simulink model "propagationSimulator"  (R2020a)
settings: Solver=VariableStepAuto  StartTime=0.0  StopTime=inf  RelTol=1e-3
InitFcn:
  | initData
values from neighbouring files (symbols this model uses):
  L = 2    [initData.m]
  N = N1*N2    (= 50)    [initData.m]    (also in populationAnimator.m = size(obj.Data.Status, 2); propagationAnimator.m = size(obj.Data.Status, 2))
  R = 0.02    [initData.m]    (also in populationAnimator.m = obj.Radius; propagationAnimator.m = obj.Radius)
  state0 = zeros(N,1)    [initData.m]
  W = 1    [initData.m]
undefined symbols (not defined in the file or in its folder): DiscIntNeverNeededParam, healTime, immobilized, pos0, v0
libraries: simulink x3
settings Model: SimulationMode=accelerator  PauseTimes=8.4  PacingRate=2  OrderedModelArguments=off  Creator=guy  LastModifiedBy=Pavel Roslovets
settings SolverCC: ZeroCrossAlgorithm=Adaptive
settings DataIOCC: MaxDataPoints=1
settings DebuggingCC: ReadBeforeWriteMsg=DisableAll  WriteAfterWriteMsg=DisableAll  WriteAfterReadMsg=DisableAll  ArithmeticOperatorsInVariantConditions=warning
settings SFSimCC: SimUseLocalCustomCode=off  CustomCodeUndefinedFunction=UseInterfaceOnly
settings RTWCC: RTWUseLocalCustomCode=off

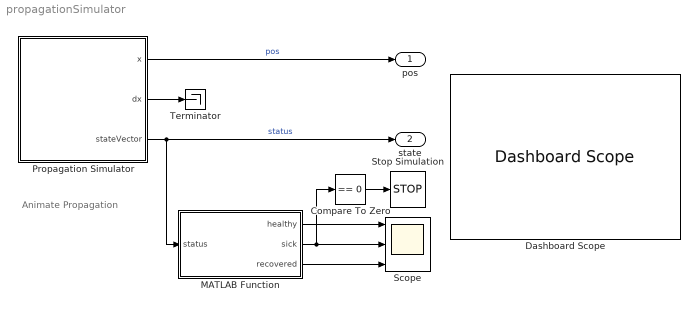
== system propagationSimulator ==
  note: Animate Propagation
  Compare To Zero : simulink/Logic and Bit Operations/Compare To Zero  relop===  OutDataTypeStr=boolean
  Dashboard Scope : DashboardScope  Ymin=0  Ymax=100
  MATLAB Function : MATLAB Function  TreatAsAtomicUnit=on
  Propagation Simulator : Stateflow chart  TreatAsAtomicUnit=on
  Scope : Scope  NumInputPorts=3
  Stop Simulation : Stop
  Terminator : Terminator
  pos : Outport  VectorParamsAs1DForOutWhenUnconnected=off
  state : Outport  Port=2  VectorParamsAs1DForOutWhenUnconnected=off
  wires:
  Propagation Simulator/1(x) -> pos/1  "pos"
  Propagation Simulator/2(dx) -> Terminator/1
  Compare To Zero/1 -> Stop Simulation/1
  MATLAB Function/1(healthy) -> Scope/1
  MATLAB Function/2(sick) -> Scope/2, Compare To Zero/1
  MATLAB Function/3(recovered) -> Scope/3
  Propagation Simulator/3(stateVector) -> state/1, MATLAB Function/1(status)  "status"

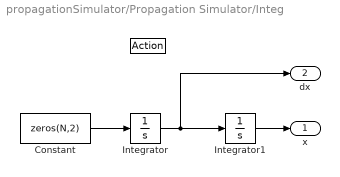
== system propagationSimulator/Propagation Simulator/Integ ==
  " " : ActionPort
      settings: CopyFcn=Stateflow.SLINSF.SimulinkMan.removeBlockPreDeleteFcn  PreDeleteFcn=Stateflow.SLINSF.SimulinkMan.unsafePredeleteFcn
  Constant : Constant  Value=zeros(N,2)
  Integrator : Integrator  ContinuousStateAttributes='dx0'
  Integrator1 : Integrator  ContinuousStateAttributes='x0'
  x : Outport  OutDataTypeStr=double  PortDimensions=[N 2]  VectorParamsAs1DForOutWhenUnconnected=off
  dx : Outport  Port=2  OutDataTypeStr=double  PortDimensions=[N 2]  VectorParamsAs1DForOutWhenUnconnected=off
  wires:
  Integrator1/1 -> x/1
  Constant/1 -> Integrator/1
  Integrator/1 -> dx/1, Integrator1/1

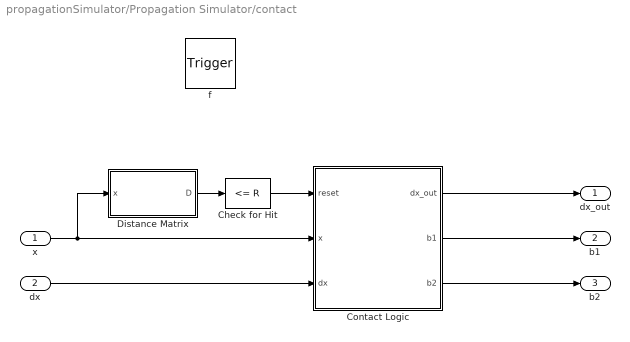
== system propagationSimulator/Propagation Simulator/contact ==
  x : Inport  OutDataTypeStr=double  PortDimensions=[N 2]
  dx : Inport  Port=2  OutDataTypeStr=double  PortDimensions=[N 2]
  f : TriggerPort  TriggerType=function-call  VariantControl=(inherit)
      settings: CopyFcn=Stateflow.SLINSF.SimulinkMan.removeBlockPreDeleteFcn  PreDeleteFcn=Stateflow.SLINSF.SimulinkMan.unsafePredeleteFcn
  Check for Hit : simulink/Logic and Bit Operations/Compare To Constant  relop=<=  const=R  OutDataTypeStr=boolean
  Contact Logic : Subsystem  TreatAsAtomicUnit=on
  Distance Matrix : Subsystem  TreatAsAtomicUnit=on
  dx_out : Outport  VectorParamsAs1DForOutWhenUnconnected=off
  b1 : Outport  Port=2
  b2 : Outport  Port=3
  wires:
  Check for Hit/1 -> Contact Logic/1(reset)
  x/1 -> Distance Matrix/1(x), Contact Logic/2(x)
  dx/1 -> Contact Logic/3(dx)
  Distance Matrix/1(D) -> Check for Hit/1
  Contact Logic/2(b1) -> b1/1
  Contact Logic/3(b2) -> b2/1
  Contact Logic/1(dx_out) -> dx_out/1

== system propagationSimulator/Propagation Simulator/heal ==
  stateIn : Inport  OutDataTypeStr=double  PortDimensions=N
  f : TriggerPort  TriggerType=function-call  VariantControl=(inherit)
      settings: CopyFcn=Stateflow.SLINSF.SimulinkMan.removeBlockPreDeleteFcn  PreDeleteFcn=Stateflow.SLINSF.SimulinkMan.unsafePredeleteFcn
  Compare To Constant2 : simulink/Logic and Bit Operations/Compare To Constant  relop=>=  const=healTime  OutDataTypeStr=boolean
  Discrete-Time Integrator : DiscreteIntegrator  SampleTime=-1  ICPrevOutput=DiscIntNeverNeededParam  ICPrevScaledInput=DiscIntNeverNeededParam
  MATLAB Function : MATLAB Function  TreatAsAtomicUnit=on
  stateVector : Outport
  wires:
  MATLAB Function/1(states) -> stateVector/1
  Discrete-Time Integrator/1 -> Compare To Constant2/1
  Compare To Constant2/1 -> MATLAB Function/2(immuned)
  stateIn/1 -> Discrete-Time Integrator/1, MATLAB Function/1("states ")

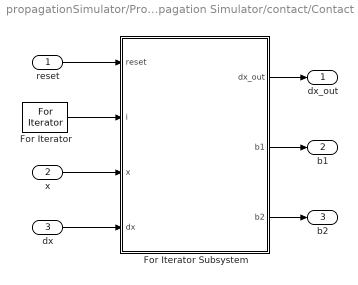
== system propagationSimulator/Propagation Simulator/contact/Contact Logic ==
  reset : Inport
  x : Inport  Port=2
  dx : Inport  Port=3
  For Iterator : ForIterator  ResetStates=reset  IterationLimit=N
  For Iterator Subsystem : Subsystem  TreatAsAtomicUnit=on
  dx_out : Outport  VectorParamsAs1DForOutWhenUnconnected=off
  b1 : Outport  Port=2
  b2 : Outport  Port=3
  wires:
  For Iterator Subsystem/1(dx_out) -> dx_out/1
  For Iterator/1 -> For Iterator Subsystem/2(i)
  reset/1 -> For Iterator Subsystem/1(reset)
  dx/1 -> For Iterator Subsystem/4(dx)
  x/1 -> For Iterator Subsystem/3(x)
  For Iterator Subsystem/2(b1) -> b1/1
  For Iterator Subsystem/3(b2) -> b2/1

== system propagationSimulator/Propagation Simulator/contact/Distance Matrix ==
  x : Inport
  For Iterator : ForIterator  ResetStates=reset  IterationLimit=N
  For Iterator Subsystem : Subsystem  TreatAsAtomicUnit=on
  D : Outport  VectorParamsAs1DForOutWhenUnconnected=off
  wires:
  For Iterator/1 -> For Iterator Subsystem/2(i)
  For Iterator Subsystem/1(Out1) -> D/1
  x/1 -> For Iterator Subsystem/1(x)

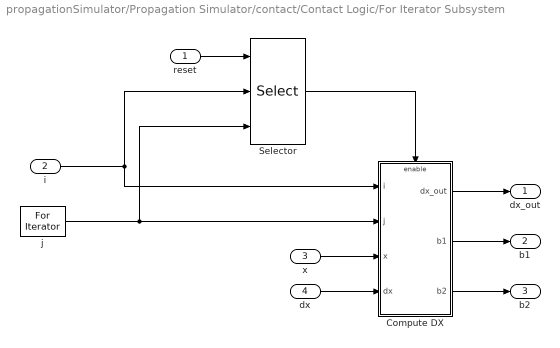
== system propagationSimulator/Propagation Simulator/contact/Contact Logic/For Iterator Subsystem ==
  reset : Inport
  i : Inport  Port=2
  x : Inport  Port=3
  dx : Inport  Port=4
  Compute DX : Subsystem
  Selector : Selector  NumberOfDimensions=2  InputPortWidth=3  IndexOptions=Index vector (port),Index vector (port)  Indices=[1 3],1  OutputSizes=1,1
  j : ForIterator  IterationLimit=N
  dx_out : Outport  VectorParamsAs1DForOutWhenUnconnected=off
  b1 : Outport  Port=2
  b2 : Outport  Port=3
  wires:
  reset/1 -> Selector/1
  j/1 -> Selector/3, Compute DX/2(j)
  i/1 -> Selector/2, Compute DX/1(i)
  Compute DX/1(dx_out) -> dx_out/1
  Selector/1 -> Compute DX/Enable
  dx/1 -> Compute DX/4(dx)
  x/1 -> Compute DX/3(x)
  Compute DX/2(b1) -> b1/1
  Compute DX/3(b2) -> b2/1

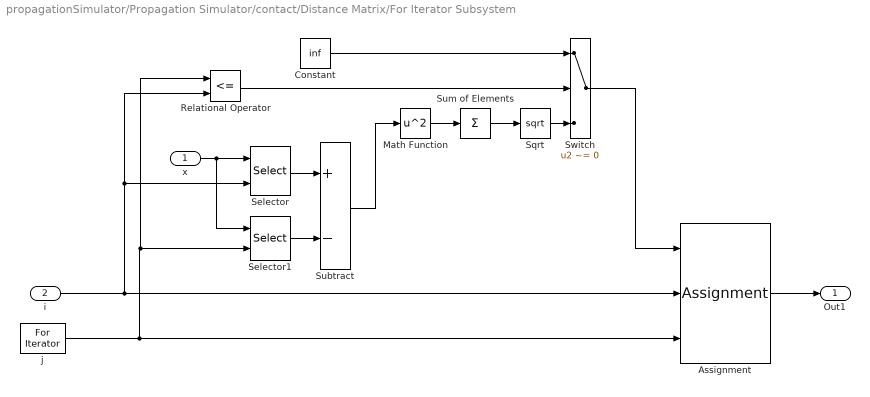
== system propagationSimulator/Propagation Simulator/contact/Distance Matrix/For Iterator Subsystem ==
  x : Inport
  i : Inport  Port=2
  Assignment : Assignment  NumberOfDimensions=2  OutputInitialize=Specify size for each dimension in table  IndexOptions=Index vector (port),Index vector (port)  Indices=1,1  OutputSizes=N,N
  Constant : Constant  Value=inf
  Math Function : Math  Operator=square  SignedPower=on  SaturateOnIntegerOverflow=on
  Relational Operator : RelationalOperator  Operator=<=  OutDataTypeStr=boolean  RndMeth=Nearest
  Selector : Selector  NumberOfDimensions=2  InputPortWidth=3  IndexOptions=Index vector (port),Select all  Indices=[1 3],1  OutputSizes=1,1
  Selector1 : Selector  NumberOfDimensions=2  InputPortWidth=3  IndexOptions=Index vector (port),Select all  Indices=[1 3],1  OutputSizes=1,1
  Sqrt : Sqrt  SaturateOnIntegerOverflow=on
  Subtract : Sum  Inputs=+-
  Sum of Elements : Sum  Inputs=+
  Switch : Switch  Criteria=u2 ~= 0
  j : ForIterator  IterationLimit=N
  Out1 : Outport  VectorParamsAs1DForOutWhenUnconnected=off
  wires:
  i/1 -> Relational Operator/2, Selector/2, Assignment/2
  j/1 -> Relational Operator/1, Selector1/2, Assignment/3
  x/1 -> Selector1/1, Selector/1
  Relational Operator/1 -> Switch/2
  Constant/1 -> Switch/1
  Selector/1 -> Subtract/1
  Selector1/1 -> Subtract/2
  Math Function/1 -> Sum of Elements/1
  Sum of Elements/1 -> Sqrt/1
  Sqrt/1 -> Switch/3
  Switch/1 -> Assignment/1
  Assignment/1 -> Out1/1
  Subtract/1 -> Math Function/1

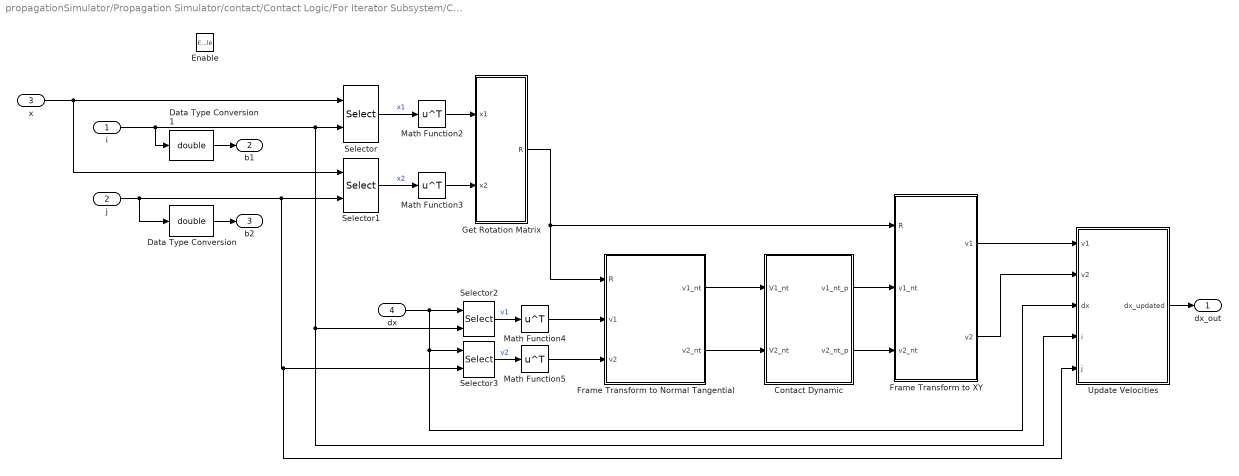
== system propagationSimulator/Propagation Simulator/contact/Contact Logic/For Iterator Subsystem/Compute DX ==
  i : Inport
  j : Inport  Port=2
  x : Inport  Port=3
  dx : Inport  Port=4
  Enable : EnablePort
  Contact Dynamic : Subsystem  Variant=on  VariantControlMode=Label  VariantControl=Choice  LabelModeActiveChoice=Simple
  Data Type Conversion : DataTypeConversion  OutDataTypeStr=double
  Data Type Conversion1 : DataTypeConversion  OutDataTypeStr=double
  Frame Transform to Normal Tangential : Subsystem
  Frame Transform to XY : Subsystem
  Get Rotation Matrix : Subsystem
  Math Function{2..5} (4 alike) : Math  Operator=transpose  SignedPower=on  SaturateOnIntegerOverflow=on
  Selector{,1..3} (4 alike) : Selector  NumberOfDimensions=2  InputPortWidth=3  IndexOptions=Index vector (port),Select all  Indices=[1 3],1  OutputSizes=1,1
  Update Velocities : Subsystem
  dx_out : Outport  VectorParamsAs1DForOutWhenUnconnected=off
  b1 : Outport  Port=2
  b2 : Outport  Port=3
  wires:
  j/1 -> Update Velocities/5(j), Selector3/2, Selector1/2, Data Type Conversion/1
  i/1 -> Update Velocities/4(i), Selector2/2, Selector/2, Data Type Conversion1/1
  Selector/1 -> Math Function2/1  "x1"
  Selector1/1 -> Math Function3/1  "x2"
  Selector2/1 -> Math Function4/1  "v1"
  Selector3/1 -> Math Function5/1  "v2"
  Update Velocities/1(dx_updated) -> dx_out/1
  Get Rotation Matrix/1(R) -> Frame Transform to Normal Tangential/1(R), Frame Transform to XY/1(R)
  Math Function2/1 -> Get Rotation Matrix/1(x1)
  Math Function3/1 -> Get Rotation Matrix/2(x2)
  Math Function4/1 -> Frame Transform to Normal Tangential/2(v1)
  Math Function5/1 -> Frame Transform to Normal Tangential/3(v2)
  Frame Transform to XY/1(v1) -> Update Velocities/1(v1)
  Frame Transform to XY/2(v2) -> Update Velocities/2(v2)
  dx/1 -> Update Velocities/3(dx), Selector3/1, Selector2/1
  x/1 -> Selector/1, Selector1/1
  Data Type Conversion/1 -> b2/1
  Data Type Conversion1/1 -> b1/1
  Frame Transform to Normal Tangential/1(v1_nt) -> Contact Dynamic/1(V1_nt)
  Frame Transform to Normal Tangential/2(v2_nt) -> Contact Dynamic/2(V2_nt)
  Contact Dynamic/2(v2_nt_p) -> Frame Transform to XY/3(v2_nt)
  Contact Dynamic/1(v1_nt_p) -> Frame Transform to XY/2(v1_nt)

== system propagationSimulator/Propagation Simulator/contact/Contact Logic/For Iterator Subsystem/Compute DX/Contact Dynamic ==
  V1_nt : Inport
  V2_nt : Inport  Port=2
  Physical model : Subsystem  VariantControl=Physical
  Simple model : Subsystem  VariantControl=Simple
  v1_nt_p : Outport
  v2_nt_p : Outport  Port=2

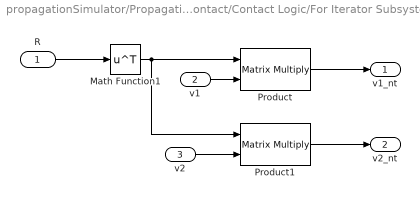
== system propagationSimulator/Propagation Simulator/contact/Contact Logic/For Iterator Subsystem/Compute DX/Frame Transform to Normal Tangential ==
  R : Inport
  v1 : Inport  Port=2
  v2 : Inport  Port=3
  Math Function1 : Math  Operator=transpose  SignedPower=on  SaturateOnIntegerOverflow=on
  Product : Product  Multiplication=Matrix(*)
  Product1 : Product  Multiplication=Matrix(*)
  v1_nt : Outport  VectorParamsAs1DForOutWhenUnconnected=off
  v2_nt : Outport  Port=2  VectorParamsAs1DForOutWhenUnconnected=off
  wires:
  v2/1 -> Product1/2
  Product/1 -> v1_nt/1
  Product1/1 -> v2_nt/1
  v1/1 -> Product/2
  Math Function1/1 -> Product1/1, Product/1
  R/1 -> Math Function1/1

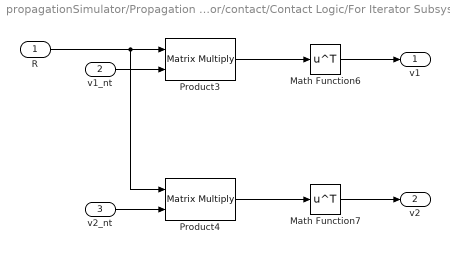
== system propagationSimulator/Propagation Simulator/contact/Contact Logic/For Iterator Subsystem/Compute DX/Frame Transform to XY ==
  R : Inport
  v1_nt : Inport  Port=2
  v2_nt : Inport  Port=3
  Math Function6 : Math  Operator=transpose  SignedPower=on  SaturateOnIntegerOverflow=on
  Math Function7 : Math  Operator=transpose  SignedPower=on  SaturateOnIntegerOverflow=on
  Product3 : Product  Multiplication=Matrix(*)
  Product4 : Product  Multiplication=Matrix(*)
  v1 : Outport  VectorParamsAs1DForOutWhenUnconnected=off
  v2 : Outport  Port=2  VectorParamsAs1DForOutWhenUnconnected=off
  wires:
  Math Function6/1 -> v1/1
  Math Function7/1 -> v2/1
  v2_nt/1 -> Product4/2
  v1_nt/1 -> Product3/2
  Product4/1 -> Math Function7/1
  Product3/1 -> Math Function6/1
  R/1 -> Product4/1, Product3/1

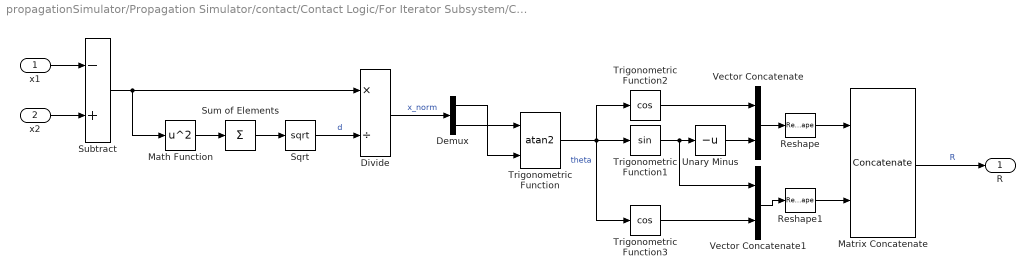
== system propagationSimulator/Propagation Simulator/contact/Contact Logic/For Iterator Subsystem/Compute DX/Get Rotation Matrix ==
  x1 : Inport
  x2 : Inport  Port=2
  Demux : Demux  Outputs=2
  Divide : Product  Inputs=*/
  Math Function : Math  Operator=square  SignedPower=on  SaturateOnIntegerOverflow=on
  Matrix Concatenate : Concatenate  Mode=Multidimensional array
  Reshape : Reshape  OutputDimensionality=Row vector (2-D)
  Reshape1 : Reshape  OutputDimensionality=Row vector (2-D)
  Sqrt : Sqrt  SaturateOnIntegerOverflow=on
  Subtract : Sum  Inputs=-+
  Sum of Elements : Sum  Inputs=+
  Trigonometric Function : Trigonometry  Operator=atan2
  Trigonometric Function1 : Trigonometry
  Trigonometric Function2 : Trigonometry  Operator=cos
  Trigonometric Function3 : Trigonometry  Operator=cos
  Unary Minus : UnaryMinus
  Vector Concatenate : Concatenate
  Vector Concatenate1 : Concatenate
  R : Outport  VectorParamsAs1DForOutWhenUnconnected=off
  wires:
  x2/1 -> Subtract/2
  Reshape1/1 -> Matrix Concatenate/2
  Trigonometric Function/1 -> Trigonometric Function3/1, Trigonometric Function1/1, Trigonometric Function2/1  "theta"
  Sum of Elements/1 -> Sqrt/1
  Subtract/1 -> Math Function/1, Divide/1
  Demux/1 -> Trigonometric Function/2
  Unary Minus/1 -> Vector Concatenate/2
  Math Function/1 -> Sum of Elements/1
  Reshape/1 -> Matrix Concatenate/1
  Matrix Concatenate/1 -> R/1  "R"
  Sqrt/1 -> Divide/2  "d"
  Trigonometric Function1/1 -> Vector Concatenate1/1, Unary Minus/1
  Vector Concatenate1/1 -> Reshape1/1
  Divide/1 -> Demux/1  "x_norm"
  Trigonometric Function2/1 -> Vector Concatenate/1
  Vector Concatenate/1 -> Reshape/1
  x1/1 -> Subtract/1
  Demux/2 -> Trigonometric Function/1
  Trigonometric Function3/1 -> Vector Concatenate1/2

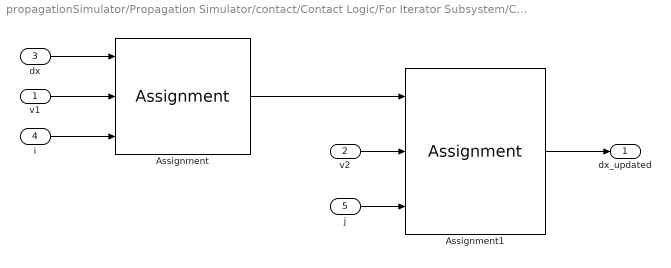
== system propagationSimulator/Propagation Simulator/contact/Contact Logic/For Iterator Subsystem/Compute DX/Update Velocities ==
  v1 : Inport
  v2 : Inport  Port=2
  dx : Inport  Port=3
  i : Inport  Port=4
  j : Inport  Port=5
  Assignment : Assignment  NumberOfDimensions=2  IndexOptions=Index vector (port),Assign all  Indices=1,1  OutputSizes=1,1
  Assignment1 : Assignment  NumberOfDimensions=2  IndexOptions=Index vector (port),Assign all  Indices=1,1  OutputSizes=1,1
  dx_updated : Outport  VectorParamsAs1DForOutWhenUnconnected=off
  wires:
  Assignment1/1 -> dx_updated/1
  Assignment/1 -> Assignment1/1
  v1/1 -> Assignment/2
  v2/1 -> Assignment1/2
  j/1 -> Assignment1/3
  i/1 -> Assignment/3
  dx/1 -> Assignment/1

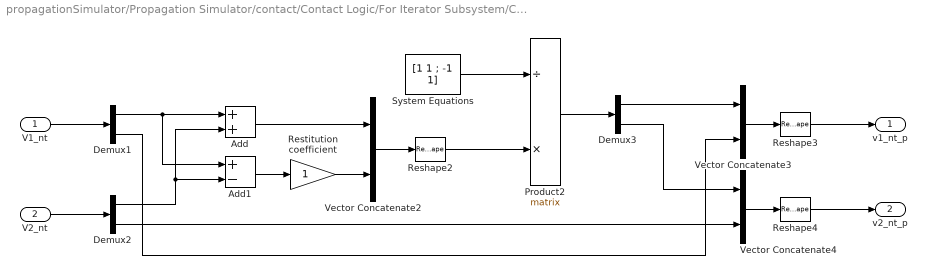
== system propagationSimulator/Propagation Simulator/contact/Contact Logic/For Iterator Subsystem/Compute DX/Contact Dynamic/Physical model ==
  V1_nt : Inport
  V2_nt : Inport  Port=2
  Add : Sum
  Add1 : Sum  Inputs=+-
  Demux1 : Demux  Outputs=2
  Demux2 : Demux  Outputs=2
  Demux3 : Demux  Outputs=2
  Product2 : Product  Inputs=/*  Multiplication=Matrix(*)
  Reshape2 : Reshape  OutputDimensionality=Column vector (2-D)
  Reshape3 : Reshape  OutputDimensionality=Column vector (2-D)
  Reshape4 : Reshape  OutputDimensionality=Column vector (2-D)
  Restitution coefficient : Gain
  System Equations : Constant  Value=[1 1 ; -1 1]
  Vector Concatenate2 : Concatenate
  Vector Concatenate3 : Concatenate
  Vector Concatenate4 : Concatenate
  v1_nt_p : Outport  VectorParamsAs1DForOutWhenUnconnected=off
  v2_nt_p : Outport  Port=2  VectorParamsAs1DForOutWhenUnconnected=off
  wires:
  Reshape4/1 -> v2_nt_p/1
  Reshape2/1 -> Product2/2
  Demux1/1 -> Add1/1, Add/1
  Restitution coefficient/1 -> Vector Concatenate2/2
  Demux2/1 -> Add1/2, Add/2
  Demux2/2 -> Vector Concatenate4/2
  Demux1/2 -> Vector Concatenate3/2
  Reshape3/1 -> v1_nt_p/1
  Product2/1 -> Demux3/1
  Vector Concatenate2/1 -> Reshape2/1
  Add/1 -> Vector Concatenate2/1
  Vector Concatenate3/1 -> Reshape3/1
  System Equations/1 -> Product2/1
  Vector Concatenate4/1 -> Reshape4/1
  Add1/1 -> Restitution coefficient/1
  V2_nt/1 -> Demux2/1
  V1_nt/1 -> Demux1/1
  Demux3/2 -> Vector Concatenate4/1
  Demux3/1 -> Vector Concatenate3/1

== system propagationSimulator/Propagation Simulator/contact/Contact Logic/For Iterator Subsystem/Compute DX/Contact Dynamic/Simple model ==
  V1_nt : Inport
  V2_nt : Inport  Port=2
  Gain1 : Gain  Gain=[-1; 1]
  Gain2 : Gain  Gain=[-1; 1]
  v1_nt_p : Outport  VectorParamsAs1DForOutWhenUnconnected=off
  v2_nt_p : Outport  Port=2  VectorParamsAs1DForOutWhenUnconnected=off
  wires:
  Gain2/1 -> v2_nt_p/1
  Gain1/1 -> v1_nt_p/1
  V2_nt/1 -> Gain2/1
  V1_nt/1 -> Gain1/1

== matlab function propagationSimulator/MATLAB Function ==
  data: status input; healthy output; sick output; recovered output
function [healthy, sick, recovered] = calc_num(status)
healthy = nnz(status == 0);
sick = nnz(status == 1);
recovered = nnz(status == 2);

== stateflow chart propagationSimulator/Propagation Simulator ==
  settings: updateMethod=CONTINUOUS
  state Integ
  state [dx_out,b1,b2] = contact(x,dx) [function]
  state stateVectorLocal = updateStatus(stateVectorLocal,bb1,bb2) [function]
    (default) -> (junction 96)
    (junction 96) -> (junction 101) [order 1] : %b1 is infected
        | [stateVectorLocal(bb1)==1]
    (junction 101) -> (junction 103) : %b2 is not
        | [stateVectorLocal(bb2)==0]
    (junction 103) -> (junction 105) : % Infect b2
        | {stateVectorLocal(bb2) = 1;}
    (junction 96) -> (junction 113) [order 2]
    (junction 113) -> (junction 109) [order 1] : %b2 is infected
        | [stateVectorLocal(bb2)==1]
    (junction 109) -> (junction 110) : %b1 is not
        | [stateVectorLocal(bb1)==0]
    (junction 113) -> (junction 115) [order 2]
    (junction 110) -> (junction 112) : % Infect b1
        | {stateVectorLocal(bb1) = 1;}
    (junction 115) -> (junction 112)
    (junction 112) -> (junction 105)
    (junction 105) -> (junction 154) : {stateVectorLocal = heal(stateVectorLocal);}
  state stateVector = heal(stateIn) [function]
  (default) -> Integ : {
      | Integ.x0 = pos0;
      | Integ.dx0 = v0;
      | stateVector = state0;
      | }
  Integ -> Integ [order 1] : [detectHit(x,dx) == true]
      | {
      | [Integ.dx0, b1, b2] = contact(x,dx);
      | stateVector = updateStatus(stateVector,b1,b2);
      | }
  Integ -> Integ [order 2] : [detectHitWall(x,dx) == true]
      | {Integ.dx0 = contactWall(x,dx);}
  data: xx function_input; hit function_output; dxx function_input; sf_internal_action_state_placeholder_data local double size=1 =0; dx0 local; x0 local; x function_input double size=[N 2]; dx function_input double size=[N 2]; dx_out function_output; b1 function_output; b2 function_output; xx function_input; dxx function_input; hitWall function_output; stateVectorLocal function_input; bb1 function_input; bb2 function_input; stateVectorLocal function_output; xx function_input; dxx function_input; dx_out function_output; stateVector function_output; stateIn function_input double size=N; x output; dx output; pos0 parameter; v0 parameter; L parameter; W parameter; R parameter; N parameter; state0 parameter; b2 local double size=1; b1 local double size=1; immobilized parameter; stateVector output =zeros(N,1)
  function hit = detectHit(xx,dxx):
    | function hit = detectHit(xx,dxx)
    |     hit = false;
    |     for i=1:size(xx, 1)
    |         % Check if two balls hit        
    |         for j=1:(i-1)
    |             dxxL = xx(i,1) - xx(j,1);
    |             dyy = xx(i,2) - xx(j,2);
    |             if sqrt(dxxL^2 + dyy^2) <= R
    |                 hit = true;
    |                 return;
    |             end
    |         end
    |     end
    | end
  function hitWall = detectHitWall(xx,dxx):
    | function hitWall = detectHitWall(xx,dxx)
    | 
    | hitWall = false;
    | for i=1:size(xx, 1)
    |     % Check if hit the wall
    |     if ((xx(i,1)>=L/2-R/2 && dxx(i,1)>0) ||...
    |             (xx(i,1)<=-L/2+R/2 && dxx(i,1)<0) ||...
    |             (xx(i,2)>=W/2-R/2 && dxx(i,2)>0) ||...
    |             (xx(i,2)<=-W/2+R/2 && dxx(i,2)<0))
    |         hitWall = true;
    |         return;
    |     end
    | end
    | end
  function dx_out = contactWall(xx,dxx):
    | function dx_out = contactWall(xx,dxx)
    | dx_out = dxx;
    | 
    | [m,~] = size(dxx);
    | 
    | % If a ball hit a wall, flip velocity sign
    | for i = 1:m
    |     
    |     if xx(i,1)>=L/2-R/2 && dxx(i,1)>0
    |         dx_out(i,1) = -dxx(i,1);
    |     end
    |     
    |     if xx(i,1)<=-L/2+R/2 && dxx(i,1)<0
    |         dx_out(i,1) = -dxx(i,1);
    |     end
    |     
    |     if xx(i,2)>=W/2-R/2 && dxx(i,2)>0
    |         dx_out(i,2) = -dxx(i,2);
    |     end
    |     
    |     if xx(i,2)<=-W/2+R/2 && dxx(i,2)<0
    |         dx_out(i,2) = -dxx(i,2);
    |     end
    |     
    | end

== matlab function propagationSimulator/Propagation Simulator/heal/MATLAB Function ==
  data: states input; states output; immuned input
function states= fcn(states, immuned)
states(immuned) = 2;
